simulink model "QuarterCarModelV2"  (R2021b)
settings: Solver=VariableStepAuto  StartTime=0.0  StopTime=3.0  RelTol=1e-3
undefined symbols (not defined in the file or in its folder): sigbuilder_block
settings Model: Creator=jpchi  LastModifiedBy=jpchi

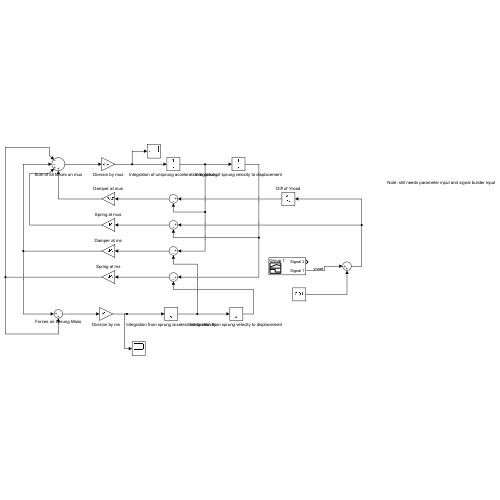
[thumbnail: Simulink's stored preview of the top-level diagram]
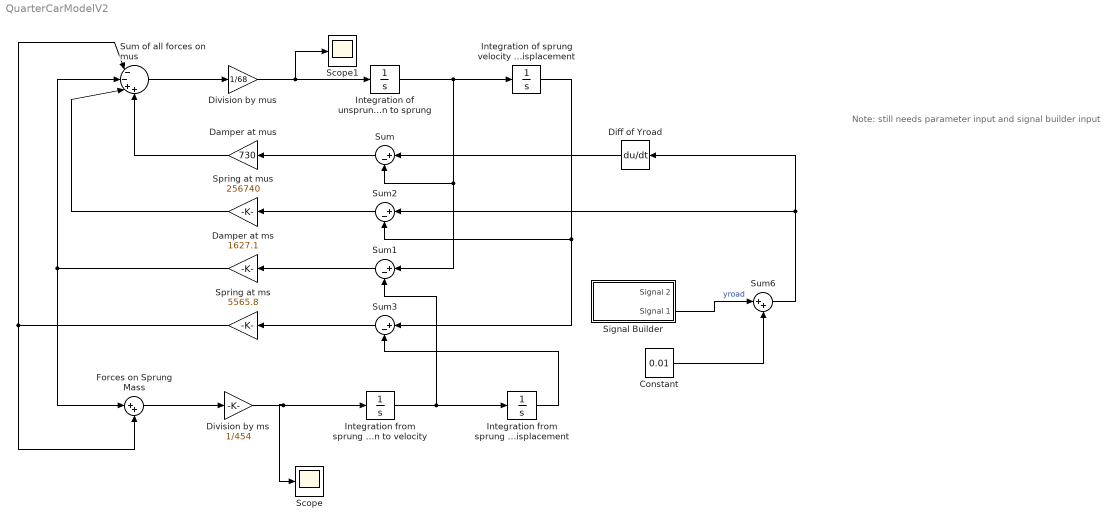
== system QuarterCarModelV2 ==
  note: Note: still needs parameter input and signal builder input
  Constant : Constant  Value=0.01
  Damper at ms : Gain  Gain=1627.1
  Damper at mus : Gain  Gain=730
  Diff of Yroad : Derivative
  Division by ms : Gain  Gain=1/454
  Division by mus : Gain  Gain=1/68
  Forces on Sprung Mass : Sum  Inputs=|++
  Integration from sprung acceleration to velocity : Integrator
  Integration from sprung velocity to displacement : Integrator
  Integration of sprung velocity to displacement : Integrator
  Integration of unsprung acceleration to sprung : Integrator
  Scope : Scope
  Scope1 : Scope
  Signal Builder : Subsystem  Tag=STV Subsys  LoadFcn=sigbuilder_block('load');  StartFcn=sigbuilder_block('start');  StopFcn=sigbuilder_block('stop');  ClipboardFcn=sigbuilder_block('clipboard');  mask(Sigbuilder block){tuvar=[0:10]}
      mask help: Simulink:masks:SigbuilderBlock_MD
      mask init:
      | if ~strcmp(get_param(bdroot(gcbh),'SimulationStatus'),'stopped') tuvar = sigbuilder_block('maskInit'); end
      settings: CopyFcn=sigbuilder_block('copy');  DeleteFcn=sigbuilder_block('delete');  ModelCloseFcn=sigbuilder_block('modelClose');  PreSaveFcn=sigbuilder_block('preSave');  PauseFcn=sigbuilder_block('pause');  ContinueFcn=sigbuilder_block('continue');  NameChangeFcn=sigbuilder_block('namechange');  OpenFcn=sigbuilder_block('open',[448.125 155.25 550.5 400.125 ]);  CloseFcn=sigbuilder_block('close');
      mask Display: plot(0, 0, 100, 100,[2, 2, 32, 32, 2], [68, 8, 8, 68, 68],[32, 2], [38, 38], [32, 19, 2],[53, 60, 44], [32, 17, 17, 2],[16, 16, 31, 31]);txt = getActiveGroup(gcbh);text(2, 100, txt,'verticalAlignment', 'top');
  Spring at ms : Gain  Gain=5565.8
  Spring at mus : Gain  Gain=256740
  Sum{,1..3} (4 alike) : Sum  Inputs=|+-
  Sum of all forces on mus : Sum  Inputs=|--++
  Sum6 : Sum  Inputs=|++
  wires:
  Constant/1 -> Sum6/2
  Signal Builder/2(Signal 1) -> Sum6/1  "yroad"
  Sum6/1 -> Sum2/1, Diff of Yroad/1
  Division by mus/1 -> Scope1/1, Integration of unsprung acceleration to sprung/1
  Integration of unsprung acceleration to sprung/1 -> Sum1/1, Sum/2, Integration of sprung velocity to displacement/1
  Integration of sprung velocity to displacement/1 -> Sum2/2, Sum3/1
  Division by ms/1 -> Scope/1, Integration from sprung acceleration to velocity/1
  Integration from sprung acceleration to velocity/1 -> Integration from sprung velocity to displacement/1, Sum1/2
  Integration from sprung velocity to displacement/1 -> Sum3/2
  Diff of Yroad/1 -> Sum/1
  Sum/1 -> Damper at mus/1
  Sum2/1 -> Spring at mus/1
  Sum1/1 -> Damper at ms/1
  Sum3/1 -> Spring at ms/1
  Spring at ms/1 -> Forces on Sprung Mass/2, Sum of all forces on mus/1
  Damper at ms/1 -> Sum of all forces on mus/2, Forces on Sprung Mass/1
  Damper at mus/1 -> Sum of all forces on mus/4
  Sum of all forces on mus/1 -> Division by mus/1
  Forces on Sprung Mass/1 -> Division by ms/1
  Spring at mus/1 -> Sum of all forces on mus/3

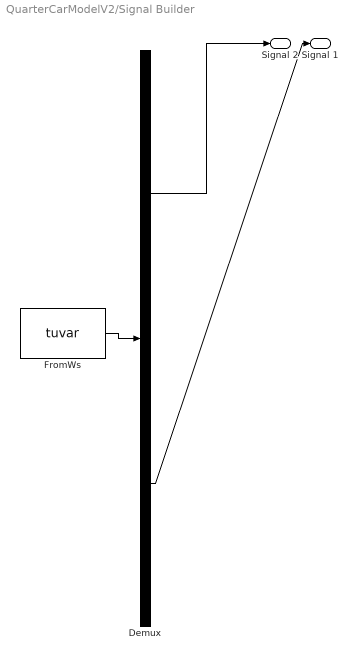
== system QuarterCarModelV2/Signal Builder ==
  Demux : Demux  Tag=STV Demux  Outputs=2
      settings: DisplayOption=none
  FromWs : FromWorkspace  Tag=STV FromWs  VariableName=tuvar
      SigBuilderData=|
      | common.afterFinalStr = 'Extrapolate'
      | common.sampleTime = 0
      | dataSet.timeRange = [0 10]
      | dataSet.name = 'Group 1'
      | sbobj.Groups.Name = 'Group 1'
      | sbobj.Groups.Signals(1).Name = 'Signal 2'
      | sbobj.Groups.Signals(1).XData = [0 1 1.05 1.1 1.15 1.2 1.21 1.25 1.27 1.3 1.35 1.4 1.45 10]
      | sbobj.Groups.Signals(1).YData = [0 0 0.014 0.042 0.098 0.35 0.35 0.166 0.126 0.09 0.052 0.022 0 0]
      | sbobj.Groups.Signals(2).Name = 'Signal 1'
      | sbobj.Groups.Signals(2).XData = [0 1 1.05 1.1 1.15 1.2 1.21 1.25 1.27 1.3 1.35 1.4 1.45 10]
      | sbobj.Groups.Signals(2).YData = [0 0 0.01 0.025 0.04 0.07 0.07 0.032 0.022 0.013 0.005 0.002 0 0]
  Signal 2 : Outport  Tag=STV Outport
  Signal 1 : Outport  Tag=STV Outport  Port=2
  wires:
  FromWs/1 -> Demux/1
  Demux/1 -> Signal 2/1
  Demux/2 -> Signal 1/1
